simulink model "ex1"  (R2020a)
settings: Solver=VariableStepAuto  StartTime=0.0  StopTime=10.0  RelTol=1e-3

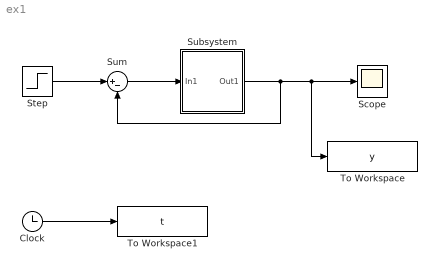
== system ex1 ==
  Clock : Clock
  Scope : Scope
  Step : Step  SampleTime=0
  Subsystem : Subsystem  mask{a=12}
      mask prompts: a "a="
      mask Callback a:
      | if str2num(get_param(gcb,'a'))<0
      |     error('Valoare negativa!')
      | end
  Sum : Sum  Inputs=|+-
  To Workspace : ToWorkspace  VariableName=y  SaveFormat=Timeseries  SampleTime=-1
  To Workspace1 : ToWorkspace  VariableName=t  SaveFormat=Timeseries  SampleTime=-1
  wires:
  Step/1 -> Sum/1
  Subsystem/1(Out1) -> Sum/2, To Workspace/1, Scope/1
  Sum/1 -> Subsystem/1(In1)
  Clock/1 -> To Workspace1/1

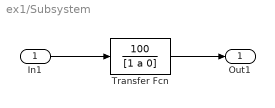
== system ex1/Subsystem ==
  In1 : Inport
  Transfer Fcn : TransferFcn  Numerator=[100]  Denominator=[1 a 0]
  Out1 : Outport
  wires:
  Transfer Fcn/1 -> Out1/1
  In1/1 -> Transfer Fcn/1
